simulink model "TST_EngReq_SmkLimCalc"  (R2016b)
settings: Solver=FixedStepDiscrete  StartTime=0.0  StopTime=simTime  FixedStep=sampleTime  RelTol=1e-3
values from neighbouring files (symbols this model uses):
  testCase = 1    [initTST_EngReq_SmkLimCalc_001.m]    (also in initTST_EngReq_SmkLimCalc_002.m = 2; initTST_EngReq_SmkLimCalc_003.m = 3)
libraries: simulink x16, UnitTest_Lib x12
settings Model: Creator=zhengjinyan  LastModifiedBy=zhengjinyan
settings DebuggingCC: SignalRangeChecking=error

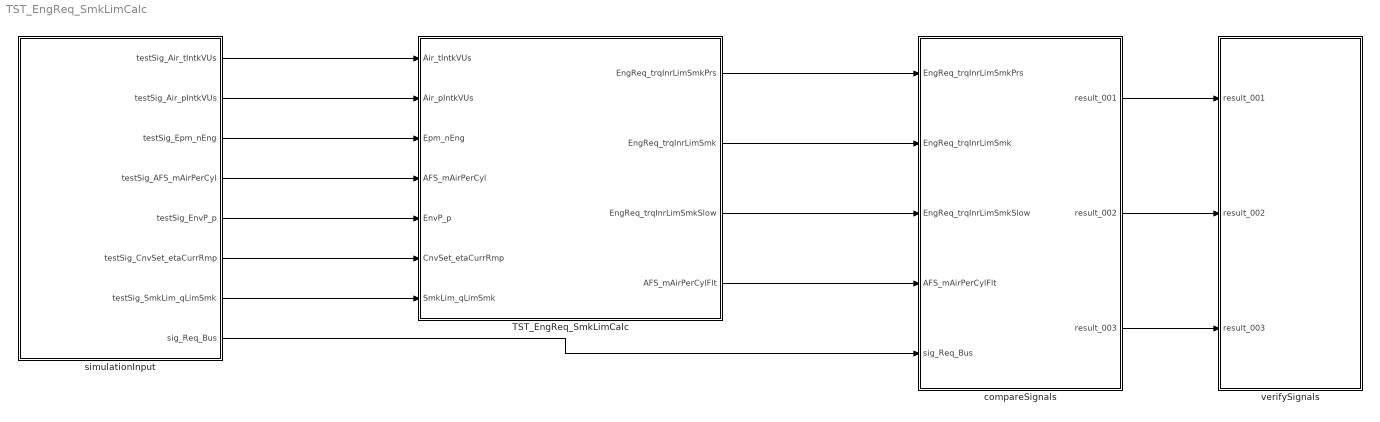
== system TST_EngReq_SmkLimCalc ==
  TST_EngReq_SmkLimCalc : Subsystem
  compareSignals : Subsystem
  simulationInput : Subsystem
  verifySignals : Subsystem
  wires:
  simulationInput/1(testSig_Air_tIntkVUs) -> TST_EngReq_SmkLimCalc/1(Air_tIntkVUs)
  simulationInput/2(testSig_Air_pIntkVUs) -> TST_EngReq_SmkLimCalc/2(Air_pIntkVUs)
  simulationInput/3(testSig_Epm_nEng) -> TST_EngReq_SmkLimCalc/3(Epm_nEng)
  simulationInput/4(testSig_AFS_mAirPerCyl) -> TST_EngReq_SmkLimCalc/4(AFS_mAirPerCyl)
  simulationInput/5(testSig_EnvP_p) -> TST_EngReq_SmkLimCalc/5(EnvP_p)
  simulationInput/6(testSig_CnvSet_etaCurrRmp) -> TST_EngReq_SmkLimCalc/6(CnvSet_etaCurrRmp)
  simulationInput/7(testSig_SmkLim_qLimSmk) -> TST_EngReq_SmkLimCalc/7(SmkLim_qLimSmk)
  TST_EngReq_SmkLimCalc/1(EngReq_trqInrLimSmkPrs) -> compareSignals/1(EngReq_trqInrLimSmkPrs)
  TST_EngReq_SmkLimCalc/2(EngReq_trqInrLimSmk) -> compareSignals/2(EngReq_trqInrLimSmk)
  TST_EngReq_SmkLimCalc/3(EngReq_trqInrLimSmkSlow) -> compareSignals/3(EngReq_trqInrLimSmkSlow)
  TST_EngReq_SmkLimCalc/4(AFS_mAirPerCylFlt) -> compareSignals/4(AFS_mAirPerCylFlt)
  simulationInput/8(sig_Req_Bus) -> compareSignals/5(sig_Req_Bus)
  compareSignals/1(result_001) -> verifySignals/1(result_001)
  compareSignals/2(result_002) -> verifySignals/2(result_002)
  compareSignals/3(result_003) -> verifySignals/3(result_003)

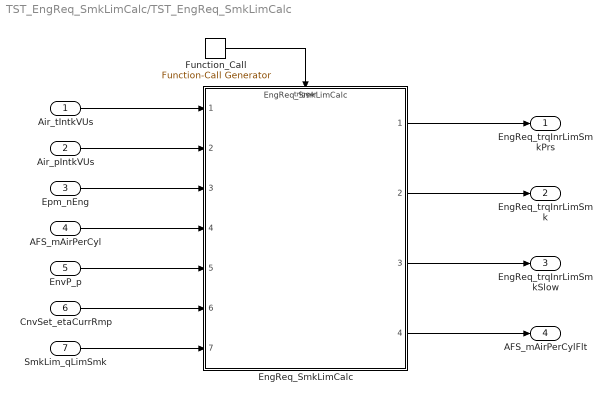
== system TST_EngReq_SmkLimCalc/TST_EngReq_SmkLimCalc ==
  Air_tIntkVUs : Inport
  Air_pIntkVUs : Inport  Port=2
  Epm_nEng : Inport  Port=3
  AFS_mAirPerCyl : Inport  Port=4
  EnvP_p : Inport  Port=5
  CnvSet_etaCurrRmp : Inport  Port=6
  SmkLim_qLimSmk : Inport  Port=7
  EngReq_SmkLimCalc : ModelReference  ModelNameDialog=EngReq_SmkLimCalc  SimulationMode=Normal  ModelReferenceVersion=1.31  TriggerPortName=function  TriggerPortTriggerType=function-call  TriggerPortStatesWhenEnabling=held
  Function_Call : simulink/Ports & Subsystems/Function-Call Generator  sample_time=sampleTime  numberOfIterations=1
  EngReq_trqInrLimSmkPrs : Outport
  EngReq_trqInrLimSmk : Outport  Port=2
  EngReq_trqInrLimSmkSlow : Outport  Port=3
  AFS_mAirPerCylFlt : Outport  Port=4
  wires:
  Function_Call/1 -> EngReq_SmkLimCalc/Trigger
  Air_tIntkVUs/1 -> EngReq_SmkLimCalc/1
  Air_pIntkVUs/1 -> EngReq_SmkLimCalc/2
  Epm_nEng/1 -> EngReq_SmkLimCalc/3
  AFS_mAirPerCyl/1 -> EngReq_SmkLimCalc/4
  EnvP_p/1 -> EngReq_SmkLimCalc/5
  CnvSet_etaCurrRmp/1 -> EngReq_SmkLimCalc/6
  SmkLim_qLimSmk/1 -> EngReq_SmkLimCalc/7
  EngReq_SmkLimCalc/1 -> EngReq_trqInrLimSmkPrs/1
  EngReq_SmkLimCalc/2 -> EngReq_trqInrLimSmk/1
  EngReq_SmkLimCalc/3 -> EngReq_trqInrLimSmkSlow/1
  EngReq_SmkLimCalc/4 -> AFS_mAirPerCylFlt/1

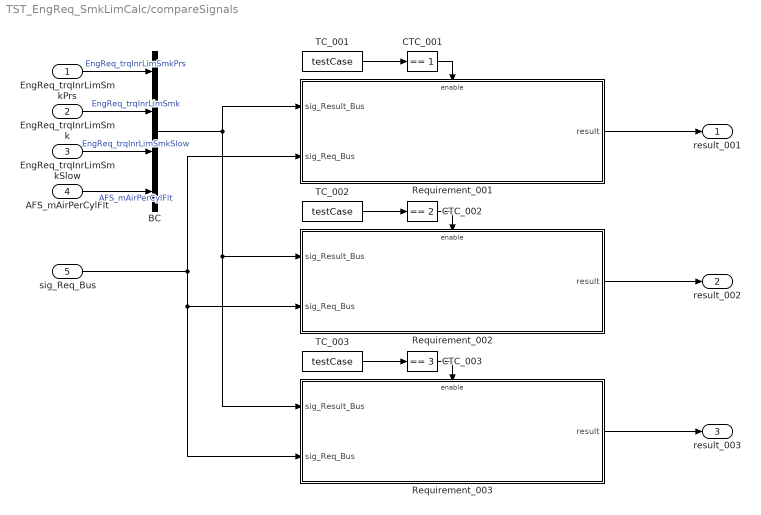
== system TST_EngReq_SmkLimCalc/compareSignals ==
  EngReq_trqInrLimSmkPrs : Inport
  EngReq_trqInrLimSmk : Inport  Port=2
  EngReq_trqInrLimSmkSlow : Inport  Port=3
  AFS_mAirPerCylFlt : Inport  Port=4
  sig_Req_Bus : Inport  Port=5
  BC : BusCreator  Inputs=4
  CTC_001 : simulink/Logic and Bit Operations/Compare To Constant  relop===  const=1  OutDataTypeStr=boolean
  CTC_002 : simulink/Logic and Bit Operations/Compare To Constant  relop===  const=2  OutDataTypeStr=boolean
  CTC_003 : simulink/Logic and Bit Operations/Compare To Constant  relop===  const=3  OutDataTypeStr=boolean
  Requirement_001 : Subsystem
  Requirement_002 : Subsystem
  Requirement_003 : Subsystem
  TC_001 : Constant  Value=testCase
  TC_002 : Constant  Value=testCase
  TC_003 : Constant  Value=testCase
  result_001 : Outport
  result_002 : Outport  Port=2
  result_003 : Outport  Port=3
  wires:
  EngReq_trqInrLimSmkPrs/1 -> BC/1  "EngReq_trqInrLimSmkPrs"
  EngReq_trqInrLimSmk/1 -> BC/2  "EngReq_trqInrLimSmk"
  EngReq_trqInrLimSmkSlow/1 -> BC/3  "EngReq_trqInrLimSmkSlow"
  AFS_mAirPerCylFlt/1 -> BC/4  "AFS_mAirPerCylFlt"
  TC_001/1 -> CTC_001/1
  CTC_001/1 -> Requirement_001/Enable
  sig_Req_Bus/1 -> Requirement_002/2(sig_Req_Bus), Requirement_003/2(sig_Req_Bus), Requirement_001/2(sig_Req_Bus)
  BC/1 -> Requirement_002/1(sig_Result_Bus), Requirement_003/1(sig_Result_Bus), Requirement_001/1(sig_Result_Bus)
  Requirement_001/1(result) -> result_001/1
  TC_002/1 -> CTC_002/1
  CTC_002/1 -> Requirement_002/Enable
  Requirement_002/1(result) -> result_002/1
  TC_003/1 -> CTC_003/1
  CTC_003/1 -> Requirement_003/Enable
  Requirement_003/1(result) -> result_003/1

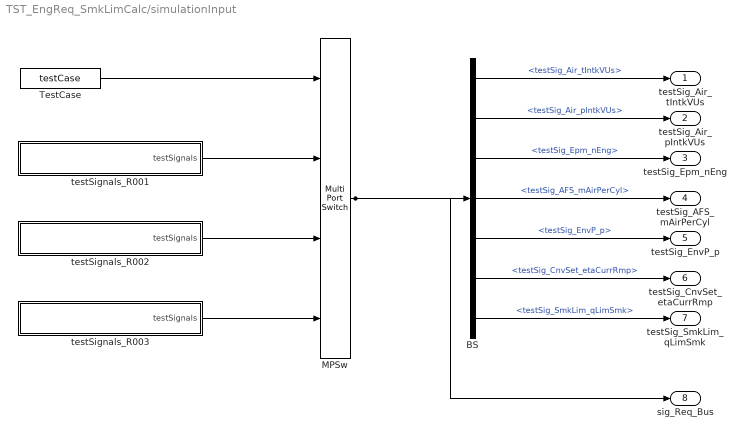
== system TST_EngReq_SmkLimCalc/simulationInput ==
  BS : BusSelector  OutputSignals=testSig_Air_tIntkVUs,testSig_Air_pIntkVUs,testSig_Epm_nEng,testSig_AFS_mAirPerCyl,testSig_EnvP_p,testSig_CnvSet_etaCurrRmp,testSig_SmkLim_qLimSmk
  MPSw : MultiPortSwitch  SaturateOnIntegerOverflow=on  InputSameDT=on
  TestCase : Constant  Value=testCase
  testSignals_R001 : Subsystem
  testSignals_R002 : Subsystem
  testSignals_R003 : Subsystem
  testSig_Air_tIntkVUs : Outport
  testSig_Air_pIntkVUs : Outport  Port=2
  testSig_Epm_nEng : Outport  Port=3
  testSig_AFS_mAirPerCyl : Outport  Port=4
  testSig_EnvP_p : Outport  Port=5
  testSig_CnvSet_etaCurrRmp : Outport  Port=6
  testSig_SmkLim_qLimSmk : Outport  Port=7
  sig_Req_Bus : Outport  Port=8
  wires:
  BS/1 -> testSig_Air_tIntkVUs/1  "<testSig_Air_tIntkVUs>"
  BS/2 -> testSig_Air_pIntkVUs/1  "<testSig_Air_pIntkVUs>"
  BS/3 -> testSig_Epm_nEng/1  "<testSig_Epm_nEng>"
  BS/4 -> testSig_AFS_mAirPerCyl/1  "<testSig_AFS_mAirPerCyl>"
  BS/5 -> testSig_EnvP_p/1  "<testSig_EnvP_p>"
  BS/6 -> testSig_CnvSet_etaCurrRmp/1  "<testSig_CnvSet_etaCurrRmp>"
  BS/7 -> testSig_SmkLim_qLimSmk/1  "<testSig_SmkLim_qLimSmk>"
  MPSw/1 -> BS/1, sig_Req_Bus/1
  TestCase/1 -> MPSw/1
  testSignals_R001/1(testSignals) -> MPSw/2
  testSignals_R002/1(testSignals) -> MPSw/3
  testSignals_R003/1(testSignals) -> MPSw/4

== system TST_EngReq_SmkLimCalc/verifySignals ==
  result_001 : Inport
  result_002 : Inport  Port=2
  result_003 : Inport  Port=3
  Assertion_001 : Assertion  Enabled=off
  Assertion_002 : Assertion  Enabled=off
  Assertion_003 : Assertion  Enabled=off
  wires:
  result_001/1 -> Assertion_001/1
  result_002/1 -> Assertion_002/1
  result_003/1 -> Assertion_003/1

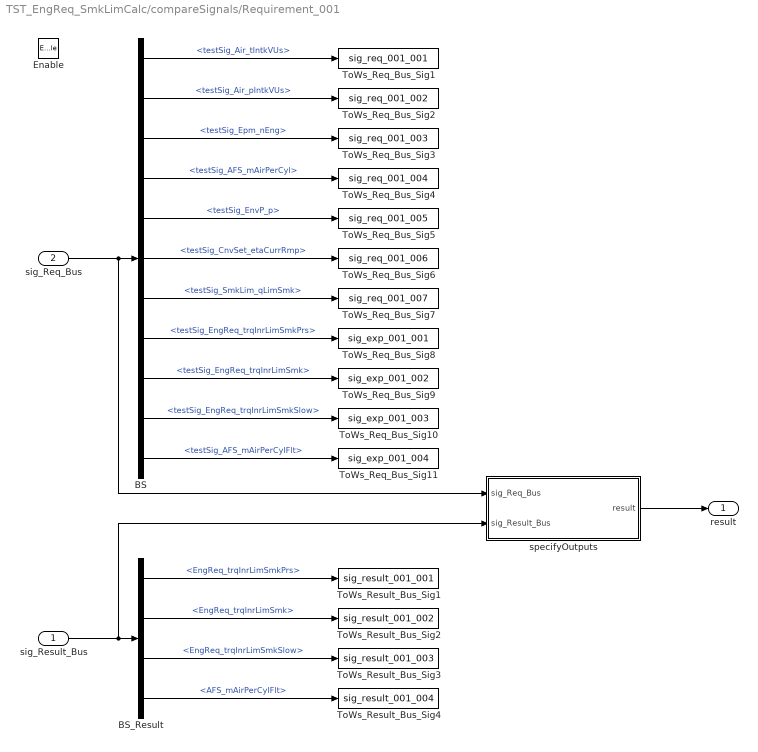
== system TST_EngReq_SmkLimCalc/compareSignals/Requirement_001 ==
  sig_Result_Bus : Inport
  sig_Req_Bus : Inport  Port=2
  Enable : EnablePort
  BS : BusSelector  OutputSignals=testSig_Air_tIntkVUs,testSig_Air_pIntkVUs,testSig_Epm_nEng,testSig_AFS_mAirPerCyl,testSig_EnvP_p,testSig_CnvSet_etaCurrRmp,testSig_SmkLim_qLimSmk,testSig_EngReq_trqInrLimSmkPrs,testSig_EngReq_trqInrLimSmk,testSig_EngReq_trqInrLimSmkSlow,testSig_AFS_mAirPerCylFlt
  BS_Result : BusSelector  OutputSignals=EngReq_trqInrLimSmkPrs,EngReq_trqInrLimSmk,EngReq_trqInrLimSmkSlow,AFS_mAirPerCylFlt
  ToWs_Req_Bus_Sig1 : ToWorkspace  VariableName=sig_req_001_001  SaveFormat=Structure With Time
  ToWs_Req_Bus_Sig10 : ToWorkspace  VariableName=sig_exp_001_003  SaveFormat=Structure With Time
  ToWs_Req_Bus_Sig11 : ToWorkspace  VariableName=sig_exp_001_004  SaveFormat=Structure With Time
  ToWs_Req_Bus_Sig2 : ToWorkspace  VariableName=sig_req_001_002  SaveFormat=Structure With Time
  ToWs_Req_Bus_Sig3 : ToWorkspace  VariableName=sig_req_001_003  SaveFormat=Structure With Time
  ToWs_Req_Bus_Sig4 : ToWorkspace  VariableName=sig_req_001_004  SaveFormat=Structure With Time
  ToWs_Req_Bus_Sig5 : ToWorkspace  VariableName=sig_req_001_005  SaveFormat=Structure With Time
  ToWs_Req_Bus_Sig6 : ToWorkspace  VariableName=sig_req_001_006  SaveFormat=Structure With Time
  ToWs_Req_Bus_Sig7 : ToWorkspace  VariableName=sig_req_001_007  SaveFormat=Structure With Time
  ToWs_Req_Bus_Sig8 : ToWorkspace  VariableName=sig_exp_001_001  SaveFormat=Structure With Time
  ToWs_Req_Bus_Sig9 : ToWorkspace  VariableName=sig_exp_001_002  SaveFormat=Structure With Time
  ToWs_Result_Bus_Sig1 : ToWorkspace  VariableName=sig_result_001_001  SaveFormat=Structure With Time
  ToWs_Result_Bus_Sig2 : ToWorkspace  VariableName=sig_result_001_002  SaveFormat=Structure With Time
  ToWs_Result_Bus_Sig3 : ToWorkspace  VariableName=sig_result_001_003  SaveFormat=Structure With Time
  ToWs_Result_Bus_Sig4 : ToWorkspace  VariableName=sig_result_001_004  SaveFormat=Structure With Time
  specifyOutputs : Subsystem
  result : Outport
  wires:
  sig_Req_Bus/1 -> BS/1, specifyOutputs/1(sig_Req_Bus)
  BS/1 -> ToWs_Req_Bus_Sig1/1  "<testSig_Air_tIntkVUs>"
  BS/2 -> ToWs_Req_Bus_Sig2/1  "<testSig_Air_pIntkVUs>"
  BS/3 -> ToWs_Req_Bus_Sig3/1  "<testSig_Epm_nEng>"
  BS/4 -> ToWs_Req_Bus_Sig4/1  "<testSig_AFS_mAirPerCyl>"
  BS/5 -> ToWs_Req_Bus_Sig5/1  "<testSig_EnvP_p>"
  BS/6 -> ToWs_Req_Bus_Sig6/1  "<testSig_CnvSet_etaCurrRmp>"
  BS/7 -> ToWs_Req_Bus_Sig7/1  "<testSig_SmkLim_qLimSmk>"
  BS/8 -> ToWs_Req_Bus_Sig8/1  "<testSig_EngReq_trqInrLimSmkPrs>"
  BS/9 -> ToWs_Req_Bus_Sig9/1  "<testSig_EngReq_trqInrLimSmk>"
  BS/10 -> ToWs_Req_Bus_Sig10/1  "<testSig_EngReq_trqInrLimSmkSlow>"
  BS/11 -> ToWs_Req_Bus_Sig11/1  "<testSig_AFS_mAirPerCylFlt>"
  sig_Result_Bus/1 -> BS_Result/1, specifyOutputs/2(sig_Result_Bus)
  BS_Result/1 -> ToWs_Result_Bus_Sig1/1  "<EngReq_trqInrLimSmkPrs>"
  BS_Result/2 -> ToWs_Result_Bus_Sig2/1  "<EngReq_trqInrLimSmk>"
  BS_Result/3 -> ToWs_Result_Bus_Sig3/1  "<EngReq_trqInrLimSmkSlow>"
  BS_Result/4 -> ToWs_Result_Bus_Sig4/1  "<AFS_mAirPerCylFlt>"
  specifyOutputs/1(result) -> result/1

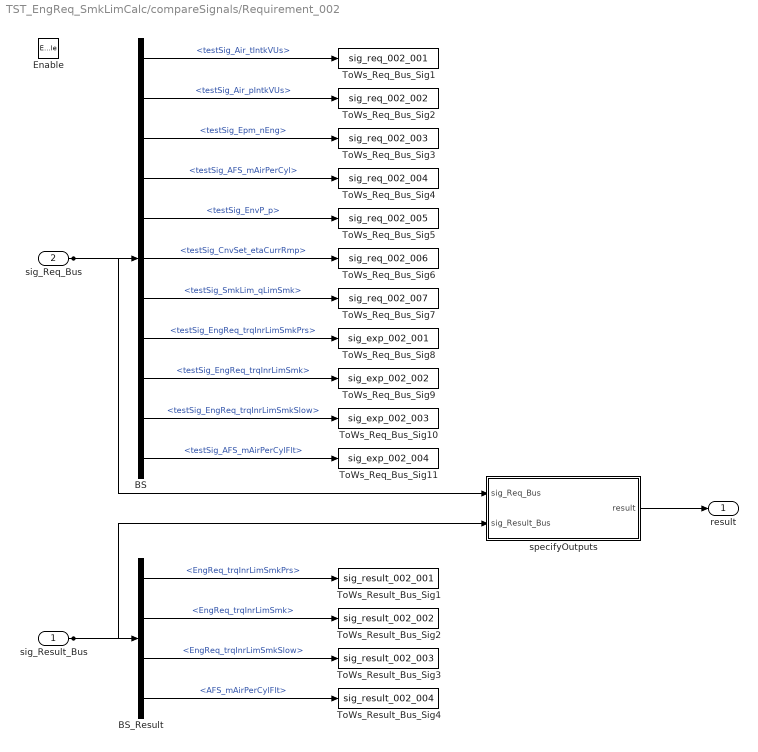
== system TST_EngReq_SmkLimCalc/compareSignals/Requirement_002 ==
  sig_Result_Bus : Inport
  sig_Req_Bus : Inport  Port=2
  Enable : EnablePort
  BS : BusSelector  OutputSignals=testSig_Air_tIntkVUs,testSig_Air_pIntkVUs,testSig_Epm_nEng,testSig_AFS_mAirPerCyl,testSig_EnvP_p,testSig_CnvSet_etaCurrRmp,testSig_SmkLim_qLimSmk,testSig_EngReq_trqInrLimSmkPrs,testSig_EngReq_trqInrLimSmk,testSig_EngReq_trqInrLimSmkSlow,testSig_AFS_mAirPerCylFlt
  BS_Result : BusSelector  OutputSignals=EngReq_trqInrLimSmkPrs,EngReq_trqInrLimSmk,EngReq_trqInrLimSmkSlow,AFS_mAirPerCylFlt
  ToWs_Req_Bus_Sig1 : ToWorkspace  VariableName=sig_req_002_001  SaveFormat=Structure With Time
  ToWs_Req_Bus_Sig10 : ToWorkspace  VariableName=sig_exp_002_003  SaveFormat=Structure With Time
  ToWs_Req_Bus_Sig11 : ToWorkspace  VariableName=sig_exp_002_004  SaveFormat=Structure With Time
  ToWs_Req_Bus_Sig2 : ToWorkspace  VariableName=sig_req_002_002  SaveFormat=Structure With Time
  ToWs_Req_Bus_Sig3 : ToWorkspace  VariableName=sig_req_002_003  SaveFormat=Structure With Time
  ToWs_Req_Bus_Sig4 : ToWorkspace  VariableName=sig_req_002_004  SaveFormat=Structure With Time
  ToWs_Req_Bus_Sig5 : ToWorkspace  VariableName=sig_req_002_005  SaveFormat=Structure With Time
  ToWs_Req_Bus_Sig6 : ToWorkspace  VariableName=sig_req_002_006  SaveFormat=Structure With Time
  ToWs_Req_Bus_Sig7 : ToWorkspace  VariableName=sig_req_002_007  SaveFormat=Structure With Time
  ToWs_Req_Bus_Sig8 : ToWorkspace  VariableName=sig_exp_002_001  SaveFormat=Structure With Time
  ToWs_Req_Bus_Sig9 : ToWorkspace  VariableName=sig_exp_002_002  SaveFormat=Structure With Time
  ToWs_Result_Bus_Sig1 : ToWorkspace  VariableName=sig_result_002_001  SaveFormat=Structure With Time
  ToWs_Result_Bus_Sig2 : ToWorkspace  VariableName=sig_result_002_002  SaveFormat=Structure With Time
  ToWs_Result_Bus_Sig3 : ToWorkspace  VariableName=sig_result_002_003  SaveFormat=Structure With Time
  ToWs_Result_Bus_Sig4 : ToWorkspace  VariableName=sig_result_002_004  SaveFormat=Structure With Time
  specifyOutputs : Subsystem
  result : Outport
  wires:
  sig_Req_Bus/1 -> BS/1, specifyOutputs/1(sig_Req_Bus)
  BS/1 -> ToWs_Req_Bus_Sig1/1  "<testSig_Air_tIntkVUs>"
  BS/2 -> ToWs_Req_Bus_Sig2/1  "<testSig_Air_pIntkVUs>"
  BS/3 -> ToWs_Req_Bus_Sig3/1  "<testSig_Epm_nEng>"
  BS/4 -> ToWs_Req_Bus_Sig4/1  "<testSig_AFS_mAirPerCyl>"
  BS/5 -> ToWs_Req_Bus_Sig5/1  "<testSig_EnvP_p>"
  BS/6 -> ToWs_Req_Bus_Sig6/1  "<testSig_CnvSet_etaCurrRmp>"
  BS/7 -> ToWs_Req_Bus_Sig7/1  "<testSig_SmkLim_qLimSmk>"
  BS/8 -> ToWs_Req_Bus_Sig8/1  "<testSig_EngReq_trqInrLimSmkPrs>"
  BS/9 -> ToWs_Req_Bus_Sig9/1  "<testSig_EngReq_trqInrLimSmk>"
  BS/10 -> ToWs_Req_Bus_Sig10/1  "<testSig_EngReq_trqInrLimSmkSlow>"
  BS/11 -> ToWs_Req_Bus_Sig11/1  "<testSig_AFS_mAirPerCylFlt>"
  sig_Result_Bus/1 -> BS_Result/1, specifyOutputs/2(sig_Result_Bus)
  BS_Result/1 -> ToWs_Result_Bus_Sig1/1  "<EngReq_trqInrLimSmkPrs>"
  BS_Result/2 -> ToWs_Result_Bus_Sig2/1  "<EngReq_trqInrLimSmk>"
  BS_Result/3 -> ToWs_Result_Bus_Sig3/1  "<EngReq_trqInrLimSmkSlow>"
  BS_Result/4 -> ToWs_Result_Bus_Sig4/1  "<AFS_mAirPerCylFlt>"
  specifyOutputs/1(result) -> result/1

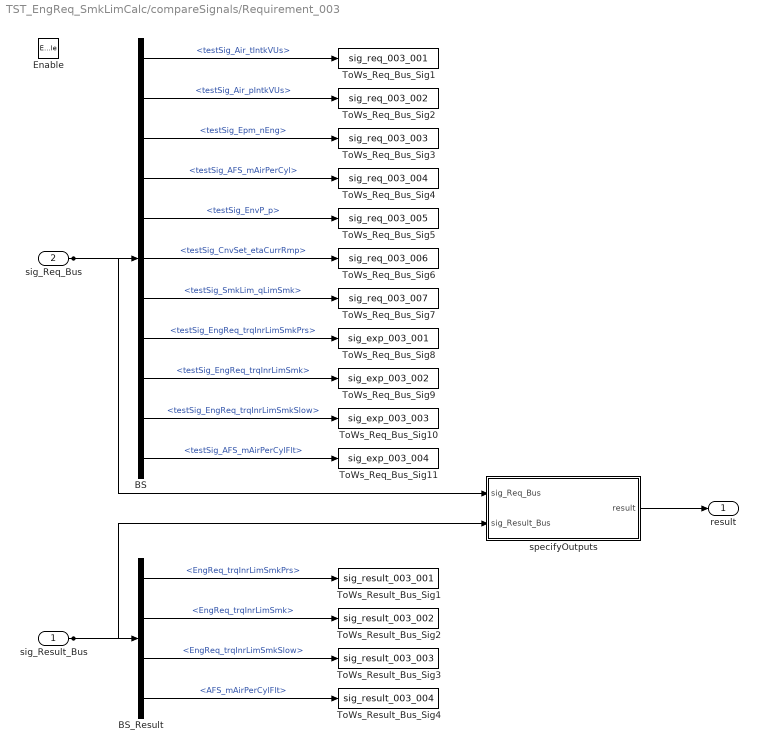
== system TST_EngReq_SmkLimCalc/compareSignals/Requirement_003 ==
  sig_Result_Bus : Inport
  sig_Req_Bus : Inport  Port=2
  Enable : EnablePort
  BS : BusSelector  OutputSignals=testSig_Air_tIntkVUs,testSig_Air_pIntkVUs,testSig_Epm_nEng,testSig_AFS_mAirPerCyl,testSig_EnvP_p,testSig_CnvSet_etaCurrRmp,testSig_SmkLim_qLimSmk,testSig_EngReq_trqInrLimSmkPrs,testSig_EngReq_trqInrLimSmk,testSig_EngReq_trqInrLimSmkSlow,testSig_AFS_mAirPerCylFlt
  BS_Result : BusSelector  OutputSignals=EngReq_trqInrLimSmkPrs,EngReq_trqInrLimSmk,EngReq_trqInrLimSmkSlow,AFS_mAirPerCylFlt
  ToWs_Req_Bus_Sig1 : ToWorkspace  VariableName=sig_req_003_001  SaveFormat=Structure With Time
  ToWs_Req_Bus_Sig10 : ToWorkspace  VariableName=sig_exp_003_003  SaveFormat=Structure With Time
  ToWs_Req_Bus_Sig11 : ToWorkspace  VariableName=sig_exp_003_004  SaveFormat=Structure With Time
  ToWs_Req_Bus_Sig2 : ToWorkspace  VariableName=sig_req_003_002  SaveFormat=Structure With Time
  ToWs_Req_Bus_Sig3 : ToWorkspace  VariableName=sig_req_003_003  SaveFormat=Structure With Time
  ToWs_Req_Bus_Sig4 : ToWorkspace  VariableName=sig_req_003_004  SaveFormat=Structure With Time
  ToWs_Req_Bus_Sig5 : ToWorkspace  VariableName=sig_req_003_005  SaveFormat=Structure With Time
  ToWs_Req_Bus_Sig6 : ToWorkspace  VariableName=sig_req_003_006  SaveFormat=Structure With Time
  ToWs_Req_Bus_Sig7 : ToWorkspace  VariableName=sig_req_003_007  SaveFormat=Structure With Time
  ToWs_Req_Bus_Sig8 : ToWorkspace  VariableName=sig_exp_003_001  SaveFormat=Structure With Time
  ToWs_Req_Bus_Sig9 : ToWorkspace  VariableName=sig_exp_003_002  SaveFormat=Structure With Time
  ToWs_Result_Bus_Sig1 : ToWorkspace  VariableName=sig_result_003_001  SaveFormat=Structure With Time
  ToWs_Result_Bus_Sig2 : ToWorkspace  VariableName=sig_result_003_002  SaveFormat=Structure With Time
  ToWs_Result_Bus_Sig3 : ToWorkspace  VariableName=sig_result_003_003  SaveFormat=Structure With Time
  ToWs_Result_Bus_Sig4 : ToWorkspace  VariableName=sig_result_003_004  SaveFormat=Structure With Time
  specifyOutputs : Subsystem
  result : Outport
  wires:
  sig_Req_Bus/1 -> BS/1, specifyOutputs/1(sig_Req_Bus)
  BS/1 -> ToWs_Req_Bus_Sig1/1  "<testSig_Air_tIntkVUs>"
  BS/2 -> ToWs_Req_Bus_Sig2/1  "<testSig_Air_pIntkVUs>"
  BS/3 -> ToWs_Req_Bus_Sig3/1  "<testSig_Epm_nEng>"
  BS/4 -> ToWs_Req_Bus_Sig4/1  "<testSig_AFS_mAirPerCyl>"
  BS/5 -> ToWs_Req_Bus_Sig5/1  "<testSig_EnvP_p>"
  BS/6 -> ToWs_Req_Bus_Sig6/1  "<testSig_CnvSet_etaCurrRmp>"
  BS/7 -> ToWs_Req_Bus_Sig7/1  "<testSig_SmkLim_qLimSmk>"
  BS/8 -> ToWs_Req_Bus_Sig8/1  "<testSig_EngReq_trqInrLimSmkPrs>"
  BS/9 -> ToWs_Req_Bus_Sig9/1  "<testSig_EngReq_trqInrLimSmk>"
  BS/10 -> ToWs_Req_Bus_Sig10/1  "<testSig_EngReq_trqInrLimSmkSlow>"
  BS/11 -> ToWs_Req_Bus_Sig11/1  "<testSig_AFS_mAirPerCylFlt>"
  sig_Result_Bus/1 -> BS_Result/1, specifyOutputs/2(sig_Result_Bus)
  BS_Result/1 -> ToWs_Result_Bus_Sig1/1  "<EngReq_trqInrLimSmkPrs>"
  BS_Result/2 -> ToWs_Result_Bus_Sig2/1  "<EngReq_trqInrLimSmk>"
  BS_Result/3 -> ToWs_Result_Bus_Sig3/1  "<EngReq_trqInrLimSmkSlow>"
  BS_Result/4 -> ToWs_Result_Bus_Sig4/1  "<AFS_mAirPerCylFlt>"
  specifyOutputs/1(result) -> result/1

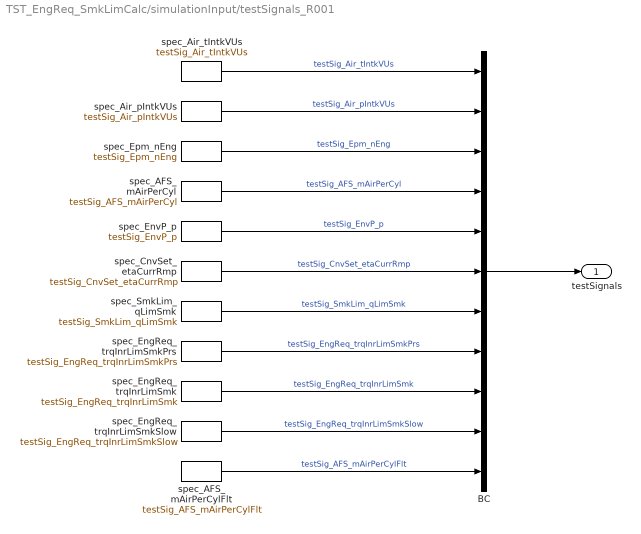
== system TST_EngReq_SmkLimCalc/simulationInput/testSignals_R001 ==
  BC : BusCreator  Inputs=11
  spec_AFS_mAirPerCyl : FromWorkspace  VariableName=testSig_AFS_mAirPerCyl  Interpolate=off  OutputAfterFinalValue=Holding final value
  spec_AFS_mAirPerCylFlt : FromWorkspace  VariableName=testSig_AFS_mAirPerCylFlt  Interpolate=off  OutputAfterFinalValue=Holding final value
  spec_Air_pIntkVUs : FromWorkspace  VariableName=testSig_Air_pIntkVUs  Interpolate=off  OutputAfterFinalValue=Holding final value
  spec_Air_tIntkVUs : FromWorkspace  VariableName=testSig_Air_tIntkVUs  Interpolate=off  OutputAfterFinalValue=Holding final value
  spec_CnvSet_etaCurrRmp : FromWorkspace  VariableName=testSig_CnvSet_etaCurrRmp  Interpolate=off  OutputAfterFinalValue=Holding final value
  spec_EngReq_trqInrLimSmk : FromWorkspace  VariableName=testSig_EngReq_trqInrLimSmk  Interpolate=off  OutputAfterFinalValue=Holding final value
  spec_EngReq_trqInrLimSmkPrs : FromWorkspace  VariableName=testSig_EngReq_trqInrLimSmkPrs  Interpolate=off  OutputAfterFinalValue=Holding final value
  spec_EngReq_trqInrLimSmkSlow : FromWorkspace  VariableName=testSig_EngReq_trqInrLimSmkSlow  Interpolate=off  OutputAfterFinalValue=Holding final value
  spec_EnvP_p : FromWorkspace  VariableName=testSig_EnvP_p  Interpolate=off  OutputAfterFinalValue=Holding final value
  spec_Epm_nEng : FromWorkspace  VariableName=testSig_Epm_nEng  Interpolate=off  OutputAfterFinalValue=Holding final value
  spec_SmkLim_qLimSmk : FromWorkspace  VariableName=testSig_SmkLim_qLimSmk  Interpolate=off  OutputAfterFinalValue=Holding final value
  testSignals : Outport
  wires:
  BC/1 -> testSignals/1
  spec_Air_tIntkVUs/1 -> BC/1  "testSig_Air_tIntkVUs"
  spec_Air_pIntkVUs/1 -> BC/2  "testSig_Air_pIntkVUs"
  spec_Epm_nEng/1 -> BC/3  "testSig_Epm_nEng"
  spec_AFS_mAirPerCyl/1 -> BC/4  "testSig_AFS_mAirPerCyl"
  spec_EnvP_p/1 -> BC/5  "testSig_EnvP_p"
  spec_CnvSet_etaCurrRmp/1 -> BC/6  "testSig_CnvSet_etaCurrRmp"
  spec_SmkLim_qLimSmk/1 -> BC/7  "testSig_SmkLim_qLimSmk"
  spec_EngReq_trqInrLimSmkPrs/1 -> BC/8  "testSig_EngReq_trqInrLimSmkPrs"
  spec_EngReq_trqInrLimSmk/1 -> BC/9  "testSig_EngReq_trqInrLimSmk"
  spec_EngReq_trqInrLimSmkSlow/1 -> BC/10  "testSig_EngReq_trqInrLimSmkSlow"
  spec_AFS_mAirPerCylFlt/1 -> BC/11  "testSig_AFS_mAirPerCylFlt"

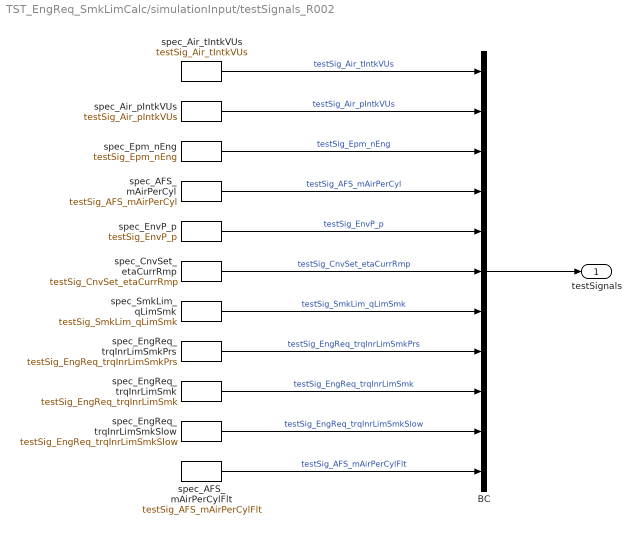
== system TST_EngReq_SmkLimCalc/simulationInput/testSignals_R002 ==
  BC : BusCreator  Inputs=11
  spec_AFS_mAirPerCyl : FromWorkspace  VariableName=testSig_AFS_mAirPerCyl  Interpolate=off  OutputAfterFinalValue=Holding final value
  spec_AFS_mAirPerCylFlt : FromWorkspace  VariableName=testSig_AFS_mAirPerCylFlt  Interpolate=off  OutputAfterFinalValue=Holding final value
  spec_Air_pIntkVUs : FromWorkspace  VariableName=testSig_Air_pIntkVUs  Interpolate=off  OutputAfterFinalValue=Holding final value
  spec_Air_tIntkVUs : FromWorkspace  VariableName=testSig_Air_tIntkVUs  Interpolate=off  OutputAfterFinalValue=Holding final value
  spec_CnvSet_etaCurrRmp : FromWorkspace  VariableName=testSig_CnvSet_etaCurrRmp  Interpolate=off  OutputAfterFinalValue=Holding final value
  spec_EngReq_trqInrLimSmk : FromWorkspace  VariableName=testSig_EngReq_trqInrLimSmk  Interpolate=off  OutputAfterFinalValue=Holding final value
  spec_EngReq_trqInrLimSmkPrs : FromWorkspace  VariableName=testSig_EngReq_trqInrLimSmkPrs  Interpolate=off  OutputAfterFinalValue=Holding final value
  spec_EngReq_trqInrLimSmkSlow : FromWorkspace  VariableName=testSig_EngReq_trqInrLimSmkSlow  Interpolate=off  OutputAfterFinalValue=Holding final value
  spec_EnvP_p : FromWorkspace  VariableName=testSig_EnvP_p  Interpolate=off  OutputAfterFinalValue=Holding final value
  spec_Epm_nEng : FromWorkspace  VariableName=testSig_Epm_nEng  Interpolate=off  OutputAfterFinalValue=Holding final value
  spec_SmkLim_qLimSmk : FromWorkspace  VariableName=testSig_SmkLim_qLimSmk  Interpolate=off  OutputAfterFinalValue=Holding final value
  testSignals : Outport
  wires:
  BC/1 -> testSignals/1
  spec_Air_tIntkVUs/1 -> BC/1  "testSig_Air_tIntkVUs"
  spec_Air_pIntkVUs/1 -> BC/2  "testSig_Air_pIntkVUs"
  spec_Epm_nEng/1 -> BC/3  "testSig_Epm_nEng"
  spec_AFS_mAirPerCyl/1 -> BC/4  "testSig_AFS_mAirPerCyl"
  spec_EnvP_p/1 -> BC/5  "testSig_EnvP_p"
  spec_CnvSet_etaCurrRmp/1 -> BC/6  "testSig_CnvSet_etaCurrRmp"
  spec_SmkLim_qLimSmk/1 -> BC/7  "testSig_SmkLim_qLimSmk"
  spec_EngReq_trqInrLimSmkPrs/1 -> BC/8  "testSig_EngReq_trqInrLimSmkPrs"
  spec_EngReq_trqInrLimSmk/1 -> BC/9  "testSig_EngReq_trqInrLimSmk"
  spec_EngReq_trqInrLimSmkSlow/1 -> BC/10  "testSig_EngReq_trqInrLimSmkSlow"
  spec_AFS_mAirPerCylFlt/1 -> BC/11  "testSig_AFS_mAirPerCylFlt"

== system TST_EngReq_SmkLimCalc/simulationInput/testSignals_R003 ==
  BC : BusCreator  Inputs=11
  spec_AFS_mAirPerCyl : FromWorkspace  VariableName=testSig_AFS_mAirPerCyl  Interpolate=off  OutputAfterFinalValue=Holding final value
  spec_AFS_mAirPerCylFlt : FromWorkspace  VariableName=testSig_AFS_mAirPerCylFlt  Interpolate=off  OutputAfterFinalValue=Holding final value
  spec_Air_pIntkVUs : FromWorkspace  VariableName=testSig_Air_pIntkVUs  Interpolate=off  OutputAfterFinalValue=Holding final value
  spec_Air_tIntkVUs : FromWorkspace  VariableName=testSig_Air_tIntkVUs  Interpolate=off  OutputAfterFinalValue=Holding final value
  spec_CnvSet_etaCurrRmp : FromWorkspace  VariableName=testSig_CnvSet_etaCurrRmp  Interpolate=off  OutputAfterFinalValue=Holding final value
  spec_EngReq_trqInrLimSmk : FromWorkspace  VariableName=testSig_EngReq_trqInrLimSmk  Interpolate=off  OutputAfterFinalValue=Holding final value
  spec_EngReq_trqInrLimSmkPrs : FromWorkspace  VariableName=testSig_EngReq_trqInrLimSmkPrs  Interpolate=off  OutputAfterFinalValue=Holding final value
  spec_EngReq_trqInrLimSmkSlow : FromWorkspace  VariableName=testSig_EngReq_trqInrLimSmkSlow  Interpolate=off  OutputAfterFinalValue=Holding final value
  spec_EnvP_p : FromWorkspace  VariableName=testSig_EnvP_p  Interpolate=off  OutputAfterFinalValue=Holding final value
  spec_Epm_nEng : FromWorkspace  VariableName=testSig_Epm_nEng  Interpolate=off  OutputAfterFinalValue=Holding final value
  spec_SmkLim_qLimSmk : FromWorkspace  VariableName=testSig_SmkLim_qLimSmk  Interpolate=off  OutputAfterFinalValue=Holding final value
  testSignals : Outport
  wires:
  BC/1 -> testSignals/1
  spec_Air_tIntkVUs/1 -> BC/1  "testSig_Air_tIntkVUs"
  spec_Air_pIntkVUs/1 -> BC/2  "testSig_Air_pIntkVUs"
  spec_Epm_nEng/1 -> BC/3  "testSig_Epm_nEng"
  spec_AFS_mAirPerCyl/1 -> BC/4  "testSig_AFS_mAirPerCyl"
  spec_EnvP_p/1 -> BC/5  "testSig_EnvP_p"
  spec_CnvSet_etaCurrRmp/1 -> BC/6  "testSig_CnvSet_etaCurrRmp"
  spec_SmkLim_qLimSmk/1 -> BC/7  "testSig_SmkLim_qLimSmk"
  spec_EngReq_trqInrLimSmkPrs/1 -> BC/8  "testSig_EngReq_trqInrLimSmkPrs"
  spec_EngReq_trqInrLimSmk/1 -> BC/9  "testSig_EngReq_trqInrLimSmk"
  spec_EngReq_trqInrLimSmkSlow/1 -> BC/10  "testSig_EngReq_trqInrLimSmkSlow"
  spec_AFS_mAirPerCylFlt/1 -> BC/11  "testSig_AFS_mAirPerCylFlt"

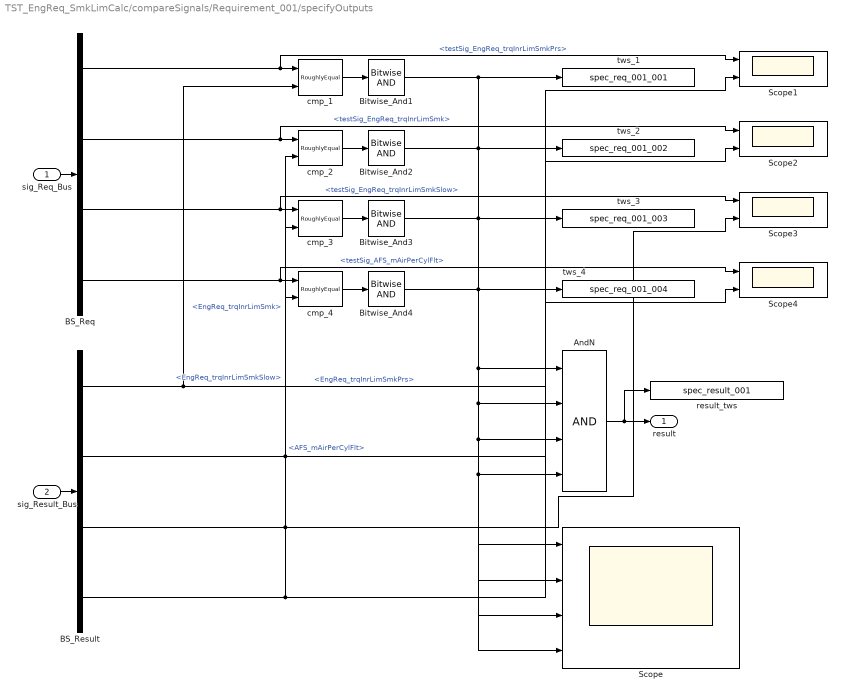
== system TST_EngReq_SmkLimCalc/compareSignals/Requirement_001/specifyOutputs ==
  sig_Req_Bus : Inport
  sig_Result_Bus : Inport  Port=2
  AndN : Logic  Inputs=4
  BS_Req : BusSelector  OutputSignals=testSig_EngReq_trqInrLimSmkPrs,testSig_EngReq_trqInrLimSmk,testSig_EngReq_trqInrLimSmkSlow,testSig_AFS_mAirPerCylFlt
  BS_Result : BusSelector  OutputSignals=EngReq_trqInrLimSmkPrs,EngReq_trqInrLimSmk,EngReq_trqInrLimSmkSlow,AFS_mAirPerCylFlt
  Bitwise_And{1..4} (4 alike) : simulink/Logic and Bit Operations/Bitwise Operator  logicop=AND  UseBitMask=off  BitMask=bin2dec('11011001')  BitMaskRealWorld=Stored Integer
  Scope : Scope  NumInputPorts=4
  Scope{1..4} (4 alike) : Scope  NumInputPorts=2
  cmp_1 : UnitTest_Lib/RoughlyEqual  slope=1
  cmp_2 : UnitTest_Lib/RoughlyEqual  slope=1
  cmp_3 : UnitTest_Lib/RoughlyEqual  slope=1
  cmp_4 : UnitTest_Lib/RoughlyEqual  slope=0.1
  result_tws : ToWorkspace  VariableName=spec_result_001
  tws_1 : ToWorkspace  VariableName=spec_req_001_001
  tws_2 : ToWorkspace  VariableName=spec_req_001_002
  tws_3 : ToWorkspace  VariableName=spec_req_001_003
  tws_4 : ToWorkspace  VariableName=spec_req_001_004
  result : Outport
  wires:
  sig_Req_Bus/1 -> BS_Req/1
  sig_Result_Bus/1 -> BS_Result/1
  AndN/1 -> result/1, result_tws/1
  BS_Req/1 -> cmp_1/1, Scope1/1  "<testSig_EngReq_trqInrLimSmkPrs>"
  BS_Result/1 -> cmp_1/2, Scope1/2  "<EngReq_trqInrLimSmkPrs>"
  cmp_1/1 -> Bitwise_And1/1
  Bitwise_And1/1 -> AndN/1, Scope/1, tws_1/1
  BS_Req/2 -> cmp_2/1, Scope2/1  "<testSig_EngReq_trqInrLimSmk>"
  BS_Result/2 -> cmp_2/2, Scope2/2  "<EngReq_trqInrLimSmk>"
  cmp_2/1 -> Bitwise_And2/1
  Bitwise_And2/1 -> AndN/2, Scope/2, tws_2/1
  BS_Req/3 -> cmp_3/1, Scope3/1  "<testSig_EngReq_trqInrLimSmkSlow>"
  BS_Result/3 -> cmp_3/2, Scope3/2  "<EngReq_trqInrLimSmkSlow>"
  cmp_3/1 -> Bitwise_And3/1
  Bitwise_And3/1 -> AndN/3, Scope/3, tws_3/1
  BS_Req/4 -> cmp_4/1, Scope4/1  "<testSig_AFS_mAirPerCylFlt>"
  BS_Result/4 -> cmp_4/2, Scope4/2  "<AFS_mAirPerCylFlt>"
  cmp_4/1 -> Bitwise_And4/1
  Bitwise_And4/1 -> AndN/4, Scope/4, tws_4/1

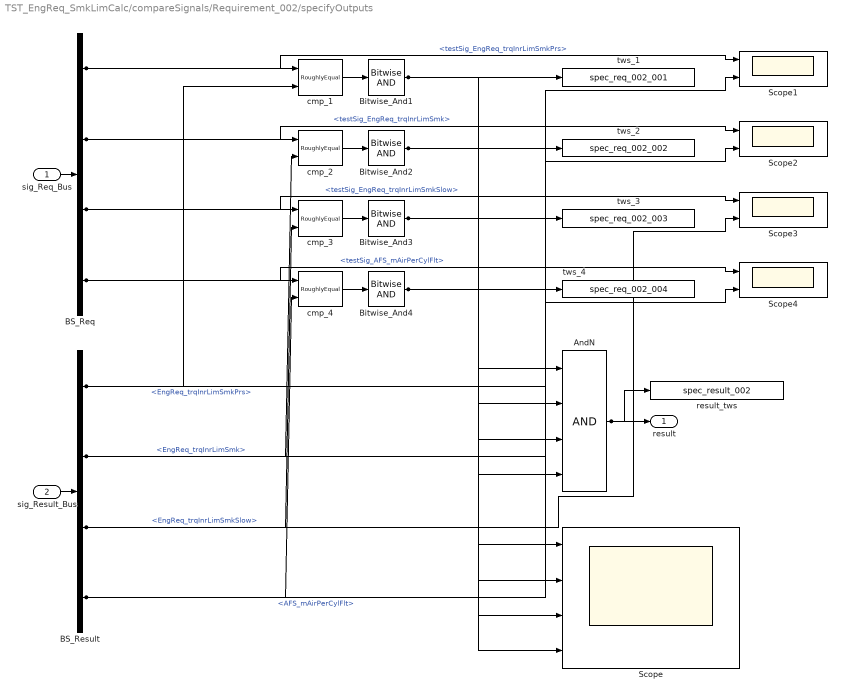
== system TST_EngReq_SmkLimCalc/compareSignals/Requirement_002/specifyOutputs ==
  sig_Req_Bus : Inport
  sig_Result_Bus : Inport  Port=2
  AndN : Logic  Inputs=4
  BS_Req : BusSelector  OutputSignals=testSig_EngReq_trqInrLimSmkPrs,testSig_EngReq_trqInrLimSmk,testSig_EngReq_trqInrLimSmkSlow,testSig_AFS_mAirPerCylFlt
  BS_Result : BusSelector  OutputSignals=EngReq_trqInrLimSmkPrs,EngReq_trqInrLimSmk,EngReq_trqInrLimSmkSlow,AFS_mAirPerCylFlt
  Bitwise_And{1..4} (4 alike) : simulink/Logic and Bit Operations/Bitwise Operator  logicop=AND  UseBitMask=off  BitMask=bin2dec('11011001')  BitMaskRealWorld=Stored Integer
  Scope : Scope  NumInputPorts=4
  Scope{1..4} (4 alike) : Scope  NumInputPorts=2
  cmp_{1..4} (4 alike) : UnitTest_Lib/RoughlyEqual  slope=0.1
  result_tws : ToWorkspace  VariableName=spec_result_002
  tws_1 : ToWorkspace  VariableName=spec_req_002_001
  tws_2 : ToWorkspace  VariableName=spec_req_002_002
  tws_3 : ToWorkspace  VariableName=spec_req_002_003
  tws_4 : ToWorkspace  VariableName=spec_req_002_004
  result : Outport
  wires:
  sig_Req_Bus/1 -> BS_Req/1
  sig_Result_Bus/1 -> BS_Result/1
  AndN/1 -> result/1, result_tws/1
  BS_Req/1 -> cmp_1/1, Scope1/1  "<testSig_EngReq_trqInrLimSmkPrs>"
  BS_Result/1 -> cmp_1/2, Scope1/2  "<EngReq_trqInrLimSmkPrs>"
  cmp_1/1 -> Bitwise_And1/1
  Bitwise_And1/1 -> tws_1/1, AndN/1, Scope/1
  BS_Req/2 -> cmp_2/1, Scope2/1  "<testSig_EngReq_trqInrLimSmk>"
  BS_Result/2 -> cmp_2/2, Scope2/2  "<EngReq_trqInrLimSmk>"
  cmp_2/1 -> Bitwise_And2/1
  Bitwise_And2/1 -> tws_2/1, AndN/2, Scope/2
  BS_Req/3 -> cmp_3/1, Scope3/1  "<testSig_EngReq_trqInrLimSmkSlow>"
  BS_Result/3 -> cmp_3/2, Scope3/2  "<EngReq_trqInrLimSmkSlow>"
  cmp_3/1 -> Bitwise_And3/1
  Bitwise_And3/1 -> tws_3/1, AndN/3, Scope/3
  BS_Req/4 -> cmp_4/1, Scope4/1  "<testSig_AFS_mAirPerCylFlt>"
  BS_Result/4 -> cmp_4/2, Scope4/2  "<AFS_mAirPerCylFlt>"
  cmp_4/1 -> Bitwise_And4/1
  Bitwise_And4/1 -> tws_4/1, AndN/4, Scope/4

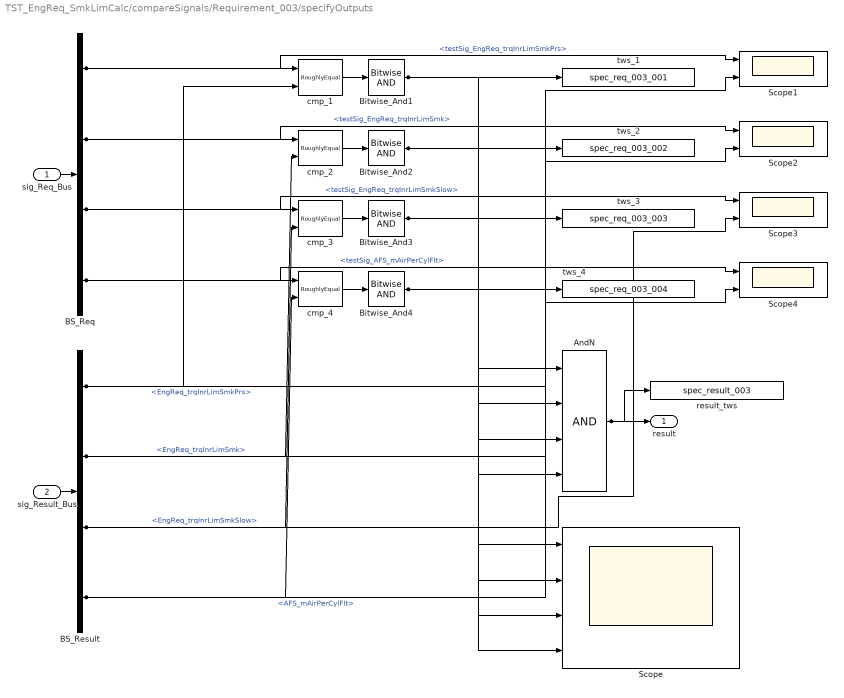
== system TST_EngReq_SmkLimCalc/compareSignals/Requirement_003/specifyOutputs ==
  sig_Req_Bus : Inport
  sig_Result_Bus : Inport  Port=2
  AndN : Logic  Inputs=4
  BS_Req : BusSelector  OutputSignals=testSig_EngReq_trqInrLimSmkPrs,testSig_EngReq_trqInrLimSmk,testSig_EngReq_trqInrLimSmkSlow,testSig_AFS_mAirPerCylFlt
  BS_Result : BusSelector  OutputSignals=EngReq_trqInrLimSmkPrs,EngReq_trqInrLimSmk,EngReq_trqInrLimSmkSlow,AFS_mAirPerCylFlt
  Bitwise_And{1..4} (4 alike) : simulink/Logic and Bit Operations/Bitwise Operator  logicop=AND  UseBitMask=off  BitMask=bin2dec('11011001')  BitMaskRealWorld=Stored Integer
  Scope : Scope  NumInputPorts=4
  Scope{1..4} (4 alike) : Scope  NumInputPorts=2
  cmp_{1..4} (4 alike) : UnitTest_Lib/RoughlyEqual  slope=0.1
  result_tws : ToWorkspace  VariableName=spec_result_003
  tws_1 : ToWorkspace  VariableName=spec_req_003_001
  tws_2 : ToWorkspace  VariableName=spec_req_003_002
  tws_3 : ToWorkspace  VariableName=spec_req_003_003
  tws_4 : ToWorkspace  VariableName=spec_req_003_004
  result : Outport
  wires:
  sig_Req_Bus/1 -> BS_Req/1
  sig_Result_Bus/1 -> BS_Result/1
  AndN/1 -> result/1, result_tws/1
  BS_Req/1 -> cmp_1/1, Scope1/1  "<testSig_EngReq_trqInrLimSmkPrs>"
  BS_Result/1 -> cmp_1/2, Scope1/2  "<EngReq_trqInrLimSmkPrs>"
  cmp_1/1 -> Bitwise_And1/1
  Bitwise_And1/1 -> tws_1/1, AndN/1, Scope/1
  BS_Req/2 -> cmp_2/1, Scope2/1  "<testSig_EngReq_trqInrLimSmk>"
  BS_Result/2 -> cmp_2/2, Scope2/2  "<EngReq_trqInrLimSmk>"
  cmp_2/1 -> Bitwise_And2/1
  Bitwise_And2/1 -> tws_2/1, AndN/2, Scope/2
  BS_Req/3 -> cmp_3/1, Scope3/1  "<testSig_EngReq_trqInrLimSmkSlow>"
  BS_Result/3 -> cmp_3/2, Scope3/2  "<EngReq_trqInrLimSmkSlow>"
  cmp_3/1 -> Bitwise_And3/1
  Bitwise_And3/1 -> tws_3/1, AndN/3, Scope/3
  BS_Req/4 -> cmp_4/1, Scope4/1  "<testSig_AFS_mAirPerCylFlt>"
  BS_Result/4 -> cmp_4/2, Scope4/2  "<AFS_mAirPerCylFlt>"
  cmp_4/1 -> Bitwise_And4/1
  Bitwise_And4/1 -> tws_4/1, AndN/4, Scope/4
